simulink model "Monitor"  (R2017b)
settings: Solver=VariableStepAuto  StartTime=0.0  StopTime=10  FixedStep=0.01  RelTol=1e-3  EnableMultiTasking=on
PreLoadFcn:
  | %Mensajes de advertencia, para que el usuario configure los parametros y el puerto antes de simular
  | disp('No olvides configurar el puerto antes de simular. Debes aclarar que puerto se usara, que velocidad y los parametros del PID.')
  | disp('A continuacion se presentan configuraciones de referencia:')
  | %Creacion de un string de parametros de referencia
  | paramString="kp_l=0.0; ki_l=0.0; td_l=0.0;"+newline,
  | %Creacion de un string de referencia que contiene el nombre del puerto
  | portString='COM3',
  | %Creacion de una variable que contiene la velocidad del puerto serie
  | serialSpeed=115200,
  | %Habilitacion de la funcion 'pause' que se utiliza en el callback 'StartFcn'
  | pause('on');
InitFcn:
  | %Creacion un objeto que permite conectarse al puerto serie, y apertura del mismo
  | serialPort=serial(portString,'BaudRate',serialSpeed);
  | fopen(serialPort);
  | %Pausa que espera a que la placa termine de configurarse luego del reinicio que ocurre cuando se abre el puerto
  | pause(3);
  | %Envio de los parametros del PID
  | fprintf(serialPort,paramString);
StopFcn:
  | %Cierre del puerto serie
  | fclose(serialPort)
libraries: LibrarySimulinkSAS x1, instrumentlib x1, sldrtlib x1, aerolibanimutils x1
CloseFcn:
  | clear portString,
  | clear paramString,
  | clear serialPort,
  | clear serialSpeed,
settings Model: SimulationMode=accelerator  Creator=Usuario  LastModifiedBy=Mauro
settings DataIOCC: LimitDataPoints=on  SaveFormat=Array
settings OptimizationCC: LifeSpan=inf
settings DebuggingCC: SolverPrmCheckMsg=warning  SFUnexpectedBacktrackingDiag=warning  SFNoUnconditionalDefaultTransitionDiag=warning  SFExecutionAtInitializationDiag=none
settings HardwareCC: ProdBitPerPointer=32  ProdBitPerSizeT=32  ProdBitPerPtrDiffT=32  ProdLargestAtomicFloat=None  ProdIntDivRoundTo=Undefined  ProdEndianess=Unspecified  ProdWordSize=32  ProdHWDeviceType=32-bit Generic
settings ModelReferenceCC: PropagateSignalLabelsOutOfModel=off
settings CodeAppCC: StateflowObjectComments=on
settings GRTTargetCC: TargetLangStandard=C89/C90 (ANSI)  GeneratePreprocessorConditionals=Disable all
settings ConfigComp: CovMetricSettings=dw  CovHtmlReporting=on  CovSaveCumulativeToWorkspaceVar=on  CovSaveSingleToWorkspaceVar=on  CovExternalEMLEnable=off  CovSFcnEnable=off

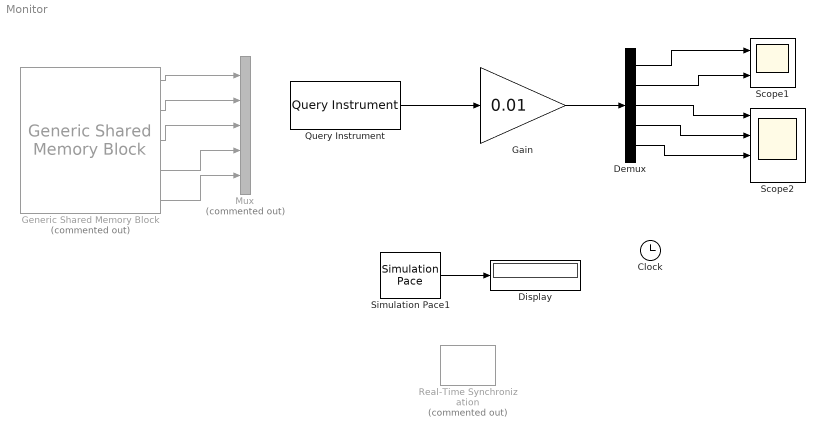
== system Monitor ==
  Clock : Clock
  Demux : Demux  Outputs=5
  Display : Display
  Gain : Gain  Gain=0.01  OutDataTypeStr=single
  Generic Shared Memory Block : LibrarySimulinkSAS/Generic Shared Memory Block  Commented=on  nombre='ARDUINO'  dispositivo=1  vecE=[34]  vecS=[1,1,1,1,1]  tipoE=['c']  tipoS=['d','d','d','d','d']  ts=0.01
      settings: SourceProductName=Library SAS
  Mux : Mux  Commented=on  Inputs=5
  Query Instrument : instrumentlib/Query Instrument  sampleTime=0.01  isWorkspaceObject=on  timeout=10  inputBufferSize=512  protocol=Serial  serialPort=COM3  baudRate=115200  gpibVendor=Agilent Technologies  boardIndex=0  primaryAddress=1  secondaryAddress=0  visaVendor=Agilent  visaSerialPort=0  chassisIndex=0  logicalAddress=0  tcpRemoteHost='127.0.0.1'  tcpRemotePort=4500  udpRemoteHost='127.0.0.1'  udpRemotePort=9090  visaTCPBoardIndex=0  visaTCPRemoteHost='127.0.0.1'  usbBoardIndex=0  usbManufID=0  usbModelCode=0  usbSerialNumber=0  wsVariableName=serialPort  initAction=None  initCommand='DATA:SOURCE CH1'  initFunction=get  queryCommand=''  responseFormat=ASCII  asciiFormatting='%d%d%d%d%d'  precision=8-bit integer  byteOrder=Little endian  valuesToRead=1  removeBytes=off  afterOutputAction=Repeat query for new data  enableFrames=on  frameSize=5
      settings: SourceProductName=Instrument Control Toolbox  SourceProductBaseCode=IC
  Real-Time Synchronization : sldrtlib/Real-Time Synchronization  Commented=on  SampleTime=0.1  MaxMissedTicks=100  ShowMissedTicks=on  YieldWhenWaiting=off
  Scope1 : Scope  NumInputPorts=2
  Scope2 : Scope  NumInputPorts=4
  Simulation Pace1 : aerolibanimutils/Simulation Pace  SimulationPace=1  SleepMode=Off  OutputPaceError=on  SampleTime=0.01
  wires:
  Demux/5 -> Scope2/3
  Demux/4 -> Scope2/2
  Demux/3 -> Scope2/1
  Demux/2 -> Scope1/2
  Demux/1 -> Scope1/1
  Simulation Pace1/1 -> Display/1
  Generic Shared Memory Block/1 -> Mux/1
  Generic Shared Memory Block/2 -> Mux/2
  Generic Shared Memory Block/3 -> Mux/3
  Generic Shared Memory Block/4 -> Mux/4
  Generic Shared Memory Block/5 -> Mux/5
  Query Instrument/1 -> Gain/1
  Gain/1 -> Demux/1
